simulink model "FullModel"  (R2024b)
settings: Solver=VariableStepAuto  StartTime=0.0  StopTime=10.0  RelTol=1e-3
settings Model: Creator=Nouran Ismail  LastModifiedBy=Nouran Ismail

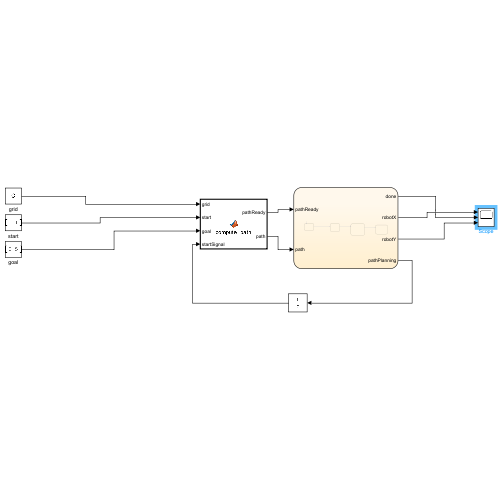
[thumbnail: Simulink's stored preview of the top-level diagram]
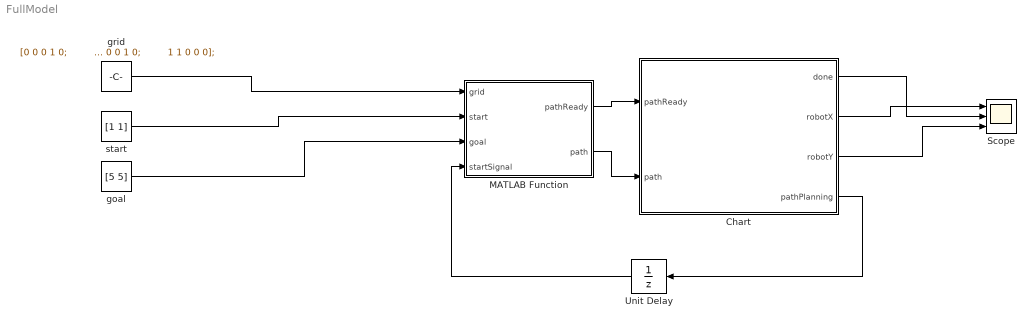
== system FullModel ==
  Chart : Stateflow chart  TreatAsAtomicUnit=on
  MATLAB Function : MATLAB Function  TreatAsAtomicUnit=on
  Scope : Scope  NumInputPorts=3
  Unit Delay : UnitDelay  SampleTime=-1  HasFrameUpgradeWarning=on
  goal : Constant  Value=[5 5]
  grid : Constant  Value=|
      | [0 0 0 1 0;
      |         0 1 0 1 0;
      |         0 1 0 0 0;
      |         0 0 0 1 0;
      |         1 1 0 0 0];
  start : Constant  Value=[1 1]
  wires:
  goal/1 -> MATLAB Function/3(goal)
  grid/1 -> MATLAB Function/1(grid)
  start/1 -> MATLAB Function/2(start)
  MATLAB Function/1(pathReady) -> Chart/1(pathReady)
  Chart/1(done) -> Scope/2
  Chart/2(robotX) -> Scope/1
  Chart/3(robotY) -> Scope/3
  Chart/4(pathPlanning) -> Unit Delay/1
  Unit Delay/1 -> MATLAB Function/4(startSignal)
  MATLAB Function/2(path) -> Chart/2(path)

== matlab function FullModel/MATLAB Function ==
  data: pathReady output; grid input; start input; path output; goal input; startSignal input
function [pathReady, path] = compute_path(grid, start, goal, startSignal)
    persistent internalPath pathFound
    
    if isempty(pathFound)
        pathFound = false;
        internalPath = zeros(size(grid));
    end

    if startSignal == 1 && ~pathFound
        rows = size(grid,1);
        cols = size(grid,2);
        current = start;
        tempPath = zeros(rows,cols);
        tempPath(current(1), current(2)) = 1;

        while ~(current(1)==goal(1) && current(2)==goal(2))
            if current(1) < goal(1)
                current(1) = current(1)+1;
            elseif current(1) > goal(1)
                current(1) = current(1)-1;
            end
            
            if current(2) < goal(2)
                current(2) = current(2)+1;
            elseif current(2) > goal(2)
                current(2) = current(2)-1;
            end
            tempPath(current(1), current(2)) = 1;
        end
        internalPath = tempPath;
        pathFound = true;
    end

    if startSignal == 0
        pathFound = false;
    end

    pathReady = pathFound;
    path = internalPath;
end

== stateflow chart FullModel/Chart ==
  state idle
    entry:
    pathPlanning= false;
  state pathPlanning
    entry:
    pathPlanning=true;
  state following
    entry:
    currentStep=1;
    during:
    if currentStep<=size(path,1)
    robotX=path(currentStep,1);
    robotY=path(currentStep,2);
    currentStep=currentStep+1;
    end
  state Goal
    entry:
    disp("Goal reached");
    done=1;
  (default) -> idle
  pathPlanning -> following : [pathReady==true]
  idle -> pathPlanning : [after(3,sec)]
  following -> Goal : [currentStep>size(path,1)]
  data: done output size=1; robotX output double size=1; robotY output double size=1; currentStep local double size=1; pathReady input boolean size=1; pathPlanning output boolean size=1; path input size=[5 5]
